simulink model "Sim_Model_2ndODE_ex4"  (Simulink 8.0)
settings: Solver=ode45  StartTime=0.0  StopTime=25  RelTol=1e-5  AbsTol=1e-8
settings Model: Creator=David  LastModifiedBy=David
settings DataIOCC: SignalLoggingSaveFormat=ModelDataLogs
settings DebuggingCC: FcnCallInpInsideContextMsg=UseLocalSettings
settings GRTTargetCC: CombineOutputUpdateFcns=off  GRTInterface=on

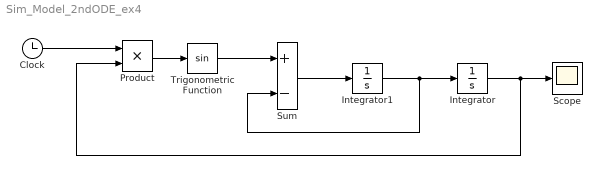
== system Sim_Model_2ndODE_ex4 ==
  Clock : Clock
  Integrator : Integrator  InitialCondition=1
  Integrator1 : Integrator  InitialCondition=2
  Product : Product  RndMeth=Zero
  Scope : Scope
  Sum : Sum  Inputs=+-
  Trigonometric Function : Trigonometry
  wires:
  Integrator1/1 -> Integrator/1, Sum/2
  Integrator/1 -> Product/2, Scope/1
  Trigonometric Function/1 -> Sum/1
  Sum/1 -> Integrator1/1
  Clock/1 -> Product/1
  Product/1 -> Trigonometric Function/1
